simulink model "robot_lego_pendule_inverse"  (R2016a)
settings: Solver=VariableStepAuto  StartTime=0.0  StopTime=10  RelTol=1e-6
undefined symbols (not defined in the file): DiscIntNeverNeededParam
libraries: simulink x1
settings Model: Creator=tmeunier  LastModifiedBy=tmeunier

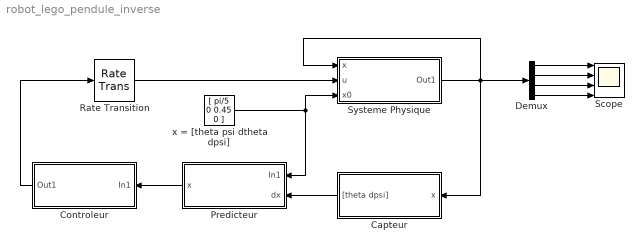
== system robot_lego_pendule_inverse ==
  Capteur : Subsystem
  Controleur : Subsystem
  Demux : Demux
  Predicteur : Subsystem
  Rate Transition : RateTransition
  Scope : Scope  NumInputPorts=4
  Systeme Physique : Subsystem
  x = [theta psi dtheta dpsi] : Constant  Value=[ pi/5 0 0.45 0 ]
  wires:
  Demux/1 -> Scope/1
  x = [theta psi dtheta dpsi]/1 -> Predicteur/1(In1), Systeme Physique/3(x0)
  Capteur/1("[theta dpsi]") -> Predicteur/2(dx)
  Systeme Physique/1(Out1) -> Capteur/1(x), Systeme Physique/1(x), Demux/1
  Controleur/1(Out1) -> Rate Transition/1
  Rate Transition/1 -> Systeme Physique/2(u)
  Predicteur/1(x) -> Controleur/1(In1)
  Demux/2 -> Scope/2
  Demux/3 -> Scope/3
  Demux/4 -> Scope/4

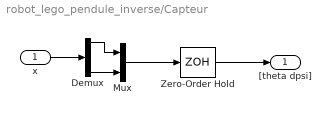
== system robot_lego_pendule_inverse/Capteur ==
  x : Inport
  Demux : Demux
  Mux : Mux  Inputs=2
  Zero-Order Hold : ZeroOrderHold  SampleTime=0.003
  "[theta dpsi]" : Outport
  wires:
  x/1 -> Demux/1
  Zero-Order Hold/1 -> "[theta dpsi]"/1
  Demux/4 -> Mux/2
  Mux/1 -> Zero-Order Hold/1
  Demux/1 -> Mux/1

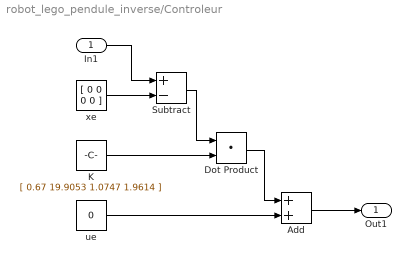
== system robot_lego_pendule_inverse/Controleur ==
  In1 : Inport
  Add : Sum
  Dot Product : DotProduct  InputSameDT=on  OutDataTypeStr=Inherit: Inherit via internal rule
  K : Constant  Value=[ 0.67 19.9053 1.0747 1.9614 ]
  Subtract : Sum  Inputs=+-
  ue : Constant  Value=0
  xe : Constant  Value=[ 0 0 0 0 ]
  Out1 : Outport
  wires:
  xe/1 -> Subtract/2
  In1/1 -> Subtract/1
  Subtract/1 -> Dot Product/1
  K/1 -> Dot Product/2
  Dot Product/1 -> Add/1
  ue/1 -> Add/2
  Add/1 -> Out1/1

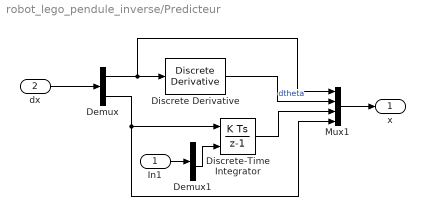
== system robot_lego_pendule_inverse/Predicteur ==
  In1 : Inport
  dx : Inport  Port=2
  Demux : Demux  Outputs=2
  Demux1 : Demux
  Discrete Derivative : simulink/Discrete/Discrete Derivative  gainval=1  ICPrevScaledInput=0.0  OutMin=[]  OutMax=[]  OutDataType=fixdt(1, 16)  OutScaling=2^-10  DoSatur=off
  Discrete-Time Integrator : DiscreteIntegrator  InitialConditionSource=external  InitialCondition=pi/10  InitialConditionSetting=State (most efficient)  SampleTime=-1  ICPrevOutput=DiscIntNeverNeededParam  ICPrevScaledInput=DiscIntNeverNeededParam
  Mux1 : Mux
  x : Outport
  wires:
  Demux1/3 -> Discrete-Time Integrator/2
  In1/1 -> Demux1/1
  dx/1 -> Demux/1
  Demux/1 -> Mux1/1, Discrete Derivative/1
  Mux1/1 -> x/1
  Demux/2 -> Mux1/4, Discrete-Time Integrator/1
  Discrete-Time Integrator/1 -> Mux1/3
  Discrete Derivative/1 -> Mux1/2  "dtheta"

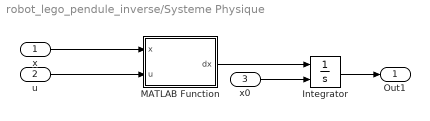
== system robot_lego_pendule_inverse/Systeme Physique ==
  x : Inport
  u : Inport  Port=2
  x0 : Inport  Port=3
  Integrator : Integrator  InitialConditionSource=external  InitialCondition=[ pi/5 0.60 ]
  MATLAB Function : MATLAB Function  TreatAsAtomicUnit=on
  Out1 : Outport
  wires:
  u/1 -> MATLAB Function/2(u)
  x/1 -> MATLAB Function/1(x)
  MATLAB Function/1(dx) -> Integrator/1
  x0/1 -> Integrator/2
  Integrator/1 -> Out1/1

== matlab function robot_lego_pendule_inverse/Systeme Physique/MATLAB Function ==
  data: x input; u input; dx output
function dx   = fonction( x, u)
%   Dynamic equations of motion of the segway on an axis.
%   Inputs: - x = [theta psi dtheta dpsi]
%               theta: average angle of the wheels      [rad]
%               psi: body pitch angle                   [rad]
%               dtheta: average velocity of the wheels  [rad/s]
%               dpsi: body pitch velocity               [rad/s]
%          - u: DC motor voltage (same value for both motors) [V]

    % State
    psi = x(2);
    dtheta = x(3);
    dpsi = x(4);

    % Parameters
    
    g = 9.81;           % gravity acceleration [m/sec^2]
    m = 0.03;           % wheel weight [kg]
    R = 0.04;           % wheel radius [m]
    Jw = m*R^2/2;       % wheel inertia moment [kg*m^2]
    M = 0.6;            % body weight [kg]
    H = 0.144;          % body height [m]
    L = H/2;            % distance of the center of mass from the wheel axle [m]
    Jpsi = M*L^2/3;     % body pitch inertia [kgm^2]
    Jm = 1e-5;          % DC motor inertia moment [kgm^2]
    Rm = 6.69;          % DC motor resistance [Ohm]
    Kb = 0.468;         % DC motor back EMF constant [Vsec/rad]
    Kt = 0.317;         % DC motor torque constant [Nm/A]
    n = 1;              % gear ratio
    fm = 0.0022;        % friction coefficient between body and DC motor
    fw = 0;             % friction coefficient between wheel and floor
    
    % Equations of motion
    c1 = (2*m+M)*R^2 + 2*Jw + 2*n^2*Jm;
    c2 = M*L*R*cos(psi) - 2*n^2*Jm;
    c3 = -M*L*R*dpsi^2*sin(psi);
    c4 = M*L^2 + Jpsi + 2*n^2*Jm;
    c5 = -M*g*L*sin(psi);

    alpha = Kt/Rm;
    beta = Kt*Kb/Rm + fm;

    Ftheta = alpha*(2*u) - 2*(beta+fw)*dtheta + 2*beta*dpsi;
    Fpsi = -alpha*(2*u) + 2*beta*dtheta - 2*beta*dpsi;

    ddtheta = (c4*c3 - c2*c5 + c4*Ftheta - c2*Fpsi)/(c4*c1 - c2^2);
    ddpsi = (Fpsi- c2*ddtheta - c5)/c4;
    dx = [dtheta dpsi ddtheta ddpsi]';

end

% Matrices of the linearized system
% E = [(2*m+M)*R^2+2*Jw+2*Jm   M*L*R-2*Jm; M*L*R-2*Jm   M*L^2+Jpsi+2*Jm];
% detE = det(E);

% alpha = Kt/Rm;
% beta = Kt*Kb/Rm + fm;

% A32 = -M*g*L*E(1,2)/detE;
% A42 = M*g*L*E(1,1)/detE;
% A33 = -(beta*E(2,2)+2*beta*E(1,2))/detE;
% A43 = (beta*E(1,2)+2*beta*E(1,1))/detE;
% A34 = beta*(E(2,2)+2*E(1,2))/detE;
% A44 = -beta*(E(1,2)+2*E(1,1))/detE;

% B3 = alpha*(E(2,2)/2+E(1,2))/detE;
% B4 = -alpha*(E(1,2)/2+E(1,1))/detE;

% A = [0 0 1 0;0 0 0 1; 0 A32 A33 A34; 0 A42 A43 A44];
% B = [0 0 2*B3 2*B4];
